simulink model "MicroMouseTemplate"  (R2024a)
settings: Solver=FixedStepAuto  StartTime=0.0  StopTime=10.0  RelTol=1e-3  EnableMultiTasking=on
undefined symbols (not defined in the file or in its folder): samplingTime
settings Model: STM32="{\"DigitalPortWrite\":[{\"ID\":\"MicroMouseTemplate:84:3\"},{\"ID\":\"MicroMouseTemplate:84:4\"},{\"ID\":\"MicroMouseTemplate:84:5\"},{\"ID\":\"MicroMouseTemplate:84:6\"},{\"ID\":\"MicroMouseTemplate:84:7\"},{\"ID\":\"MicroMouseTemplate:84:8\"},{\"ID\":\"MicroMouseTemplate:84:9\"},{\"ID\":\"MicroMouseTemplate:84:10\"},{\"ID\":\"MicroMouseTemplate:160:19\"},{\"ID\":\"MicroMouseTemplate:2479:4\"},{\"ID\":\"MicroMouseTemplate:2479:6\"},{\"ID\":\"MicroMouseTemplate:2479:7\"},{\"ID\":\"MicroMouseTemplate:2479:8\"}],\"PWMOutput\":[{\"ID\":\"MicroMouseTemplate:160:24\"},{\"ID\":\"MicroMouseTemplate:160:25\"}],\"AnalogInput\":{\"ID\":\"MicroMouseTemplate:2357:1\"},\"DigitalPortRead\":[{\"ID\":\"MicroMouseTemplate:2483:3\"},{\"ID\":\"MicroMouseTemplate:2483:4\"}]}"  SimulationMode=external  ExtModeTrigDuration=10  Creator=JesseJabezArendse  LastModifiedBy=Chris Scheepers
settings SolverCC: AllowMultiTaskInputOutput=on  AutoInsertRateTranBlk=on  InsertRTBMode=Never (minimum delay)
settings OptimizationCC: EnhancedBackFolding=on  PassReuseOutputArgsAs=Individual arguments  StateBitsets=on  DataBitsets=on  ZeroExternalMemoryAtStartup=off  ZeroInternalMemoryAtStartup=off  NoFixptDivByZeroProtection=on  MaxStackSize=64  OptimizeBlockOrder=speed  DifferentSizesBufferReuse=on  EfficientTunableParamExpr=on
settings DebuggingCC: MultiTaskCondExecSysMsg=none  ParameterOverflowMsg=none  ParameterPrecisionLossMsg=none  ParameterTunabilityLossMsg=error
settings HardwareCC: ProdBitPerPointer=32  ProdBitPerSizeT=32  ProdBitPerPtrDiffT=32  ProdLargestAtomicInteger=Long  ProdLargestAtomicFloat=Double  ProdWordSize=32  ProdLongLongMode=on  ProdHWDeviceType=ARM Compatible->ARM Cortex  TargetBitPerPointer=64  TargetBitPerSizeT=64  TargetBitPerPtrDiffT=64  TargetLongLongMode=on  TargetIntDivRoundTo=Zero  TargetEndianess=LittleEndian  TargetWordSize=64  TargetHWDeviceType=MATLAB Host
settings ModelReferenceCC: EnableParallelModelReferenceBuilds=on  ParallelModelReferenceMATLABWorkerInit=Copy Base Workspace  SupportModelReferenceSimTargetCustomCode=on
settings SFSimCC: MATLABDynamicMemAlloc=off  SimHardwareAcceleration=native
settings RTWCC: Description=Embedded Coder  SystemTargetFile=ert.tlc  HardwareBoard=STM32L4xx Based  TLCOptions=-p0 -aInlineSetEventsForThisBaseRateFcn=TLC_FALSE -aSuppressMultiTaskScheduler=TLC_FALSE -aRateBasedStepFcn=1  TemplateMakefile=ert_default_tmf  Toolchain=GNU Tools for ARM Embedded Processors  CodeExecutionProfiling=on  CodeProfilingInstrumentation=coarse  GPUComputeCapability=3.5
settings RTWCC: CustomHeaderCode=|
  | #include "MicroMouseProgramming\Core\Inc\IMU.h"
  | #include "MicroMouseProgramming\Core\Inc\CustomWhile.h"
  | #include "MicroMouseProgramming\Core\Inc\Motors.h"
settings RTWCC: CustomInclude=|
  | MicroMouseProgramming\Core\Inc\
  | MicroMouseProgramming\Core\Src\
settings RTWCC: CustomSource=|
  | MicroMouseProgramming\Core\Src\IMU.c
  | MicroMouseProgramming\Core\Src\CustomWhile.c
  | MicroMouseProgramming\Core\Src\Motors.c
settings CodeAppCC: ForceParamTrailComments=on  IgnoreCustomStorageClasses=off  OperatorAnnotations=on  SimulinkDataObjDesc=on  SFDataObjDesc=on  InsertBlockDesc=on
settings ERTTargetCC: CodeReplacementLibrary=ARM Cortex-M  SupportNonFinite=off  SupportComplex=off  SupportContinuousTime=on  ExtModeTransport=3  ExtModeStaticAlloc=on  ExtModeStaticAllocSize=2048  ExtModeMexFile=ext_xcp  ExtModeIntrfLevel=Level2 - Open

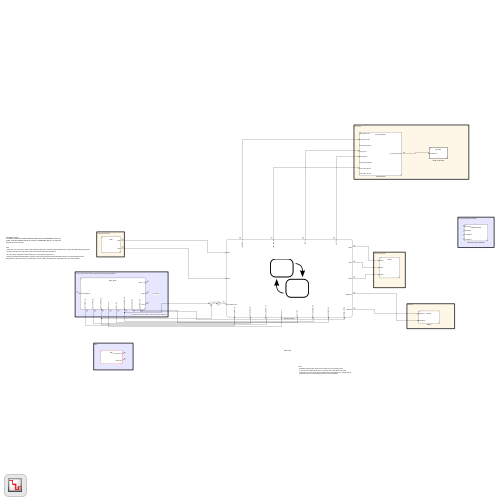
[thumbnail: Simulink's stored preview of the top-level diagram]
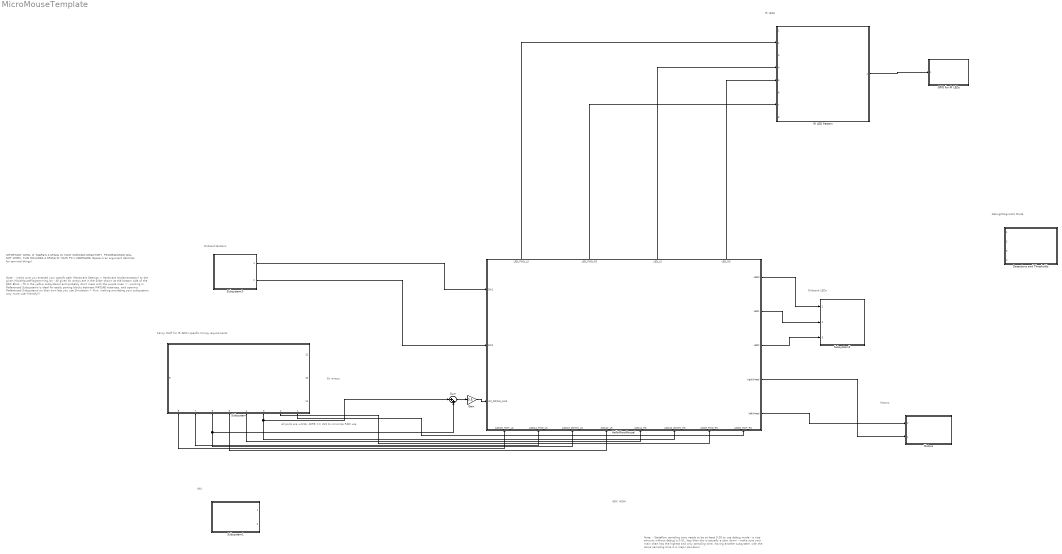
== system MicroMouseTemplate ==
  note: ADC HIGH
  note: IMPORTANT NOTE:
      | IF THERE'S A SPACE IN YOUR WORKING DIRECTORY, PROGRAMMING WILL NOT WORK, THIS INCLUDES A SPACE IN YOUR PC's USERNAME (Space is an argument delimiter for terminal things)
  note: Note:
      | - make sure you entered your specifc path (Hardware Settings > Hardware Implementation) to the given MicroMouseProgramming.ioc
      | - All given 8x arrays are in the order shown at the bottom side of the ADC Block
      |
      | - fill in the yellow subsystems and probably don't mess with the purple ones :)
      | - working in Referenced Subsystems is ideal for easily porting blocks between MATLAB instances, and opening Referenced Subsystems on their own lets you use Simulation > Run, making simulating your subsystems way more user friendly!!!
  note: 8x arrays
  note: all ports are uint16, 4095 == 3V3 to minimize RAM use
  note: IMU
  note: Note:
      | - Stateflow sampling time needs to be at least 0.05 to use debug mode
      | - a nice amount without debug is 0.01, less than this is actually a slow down
      | - make sure your main chart has the highest and only sampling time, having another
      | subsystem with the same sampling time is a major slowdown
  note: Fancy Stuff for IR ADCs specific timing requirements
  note: IR LEDs
  note: Motors
  note: Onboard Buttons
  note: Onboard LEDs
  note: Debug/Diagnostic Mode
  Detections and Thresholds : Subsystem  ReferencedSubsystem=DiagnosticMode
  GPIO for IR LEDs : Subsystem  TreatAsAtomicUnit=on  SystemSampleTime=samplingTime  ReferencedSubsystem=IR_LEDs
  Gain : Gain  Gain=0.5
  HelloMicroMouse! : Stateflow chart  TreatAsAtomicUnit=on  SystemSampleTime=0.05
      settings: PortSchema="{\"entries\":[{\"content\":{\"sides\":[{\"content\":{\"connectorIds\":[\"In11\",\"In10\",\"In3\"]},\"type\":\"ConnectorPlacement.EquallySpacedRectSide\",\"uuid\":\"f52daa4f-6374-42e5-9ef1-0ccc99d09b58\"},{\"content\":{\"connectorIds\":[\"Out5\",\"Out3\",\"Out4\",\"Out2\",\"Out1\"],\"side\":\"RIGHT\"},\"type\":\"ConnectorPlacement.EquallySpacedRectSide\",\"uuid\":\"94b478cc-4dde-45c7-a588-77cf2b43cdb7\"},{\"content\":{\"connectorIds\":[\"Out6\",\"Out7\",\"Out8\",\"Out9\"],\"side\":\"TOP\"},\"type\":\"ConnectorPlacement.EquallySpacedRectSide\",\"uuid\":\"afff2079-ea5c-423e-9722-09c3bbce433b\"},{\"content\":{\"connectorIds\":[\"In1\",\"In2\",\"In4\",\"In5\",\"In6\",\"In7\",\"In8\",\"In9\"],\"side\":\"BOTTOM\"},\"type\":\"ConnectorPlacement.EquallySpacedRectSide\",\"uuid\":\"94e93a1d-795d-41a3-b2d8-d520b2bf47ef\"}]},\"type\":\"ConnectorPlacement.EquallySpacedConnector\",\"uuid\":\"d4d35636-54af-48ac-af70-d56caef5e090\"}],\"packageUris\":[\"http://schema.mathworks.com/mf0/Connector/R2020b\"],\"version\":\"1.0\"}"
  IR LED Pattern : Subsystem  ReferencedSubsystem=IR_LED_Pattern
  Motors : Subsystem  ReferencedSubsystem=Motors
      settings: PortSchema="{\"entries\":[{\"content\":{\"sides\":[{\"content\":{\"connectorIds\":[\"In2\",\"In1\"]},\"type\":\"ConnectorPlacement.EquallySpacedRectSide\",\"uuid\":\"b3741f01-871a-479c-9206-f0581f668097\"},{\"content\":{\"side\":\"RIGHT\"},\"type\":\"ConnectorPlacement.EquallySpacedRectSide\",\"uuid\":\"4e24163a-f10e-40fa-a35f-86add3e4876d\"},{\"content\":{\"side\":\"TOP\"},\"type\":\"ConnectorPlacement.EquallySpacedRectSide\",\"uuid\":\"20b900cb-8f31-42f3-9ac1-0d679ccd8bc0\"}]},\"type\":\"ConnectorPlacement.EquallySpacedConnector\",\"uuid\":\"90358f46-f7a9-48cf-9149-c68081c17f53\"}],\"packageUris\":[\"http://schema.mathworks.com/mf0/Connector/R2020b\"],\"version\":\"1.0\"}"
  Subsystem : Subsystem  ReferencedSubsystem=ADC_Block
      settings: PortSchema="{\"entries\":[{\"content\":{\"sides\":[{\"content\":{},\"type\":\"ConnectorPlacement.EquallySpacedRectSide\",\"uuid\":\"be6b81d5-7a49-4e34-b35f-0c07892094fc\"},{\"content\":{\"connectorIds\":[\"Out1\",\"Out2\",\"Out3\",\"Out4\",\"Out5\",\"Out6\",\"Out7\",\"Out8\"],\"side\":\"RIGHT\"},\"type\":\"ConnectorPlacement.EquallySpacedRectSide\",\"uuid\":\"5e22590a-b7c0-4c63-8de4-8d81fd6c3849\"},{\"content\":{\"connectorIds\":[\"Out12\",\"Out10\",\"Out11\"],\"side\":\"TOP\"},\"type\":\"ConnectorPlacement.EquallySpacedRectSide\",\"uuid\":\"da97636e-cea0-4a10-8fe5-d807f9ee999f\"},{\"content\":{\"connectorIds\":[\"Out9\"],\"side\":\"BOTTOM\"},\"type\":\"ConnectorPlacement.EquallySpacedRectSide\",\"uuid\":\"a593d780-81a8-4730-a8bc-2bbf356cafe4\"}]},\"type\":\"ConnectorPlacement.EquallySpacedConnector\",\"uuid\":\"0bcac921-e51a-4437-9183-315712d0a8c2\"}],\"packageUris\":[\"http://schema.mathworks.com/mf0/Connector/R2020b\"],\"version\":\"1.0\"}"
  Subsystem1 : Subsystem  ReferencedSubsystem=IMU
  Subsystem2 : Subsystem  ReferencedSubsystem=LEDs
  Subsystem3 : Subsystem  ReferencedSubsystem=SWs
  Sum : Sum  Inputs=|++
  wires:
  IR LED Pattern/1 -> GPIO for IR LEDs/1
  Subsystem3/1 -> HelloMicroMouse!/11(SW1)
  HelloMicroMouse!/5(LED0) -> Subsystem2/1
  HelloMicroMouse!/3(LED1) -> Subsystem2/2
  HelloMicroMouse!/4(LED2) -> Subsystem2/3
  Sum/1 -> Gain/1
  Gain/1 -> HelloMicroMouse!/3(init_DOWN_AVG)
  Subsystem3/2 -> HelloMicroMouse!/10(SW2)
  Subsystem/1 -> HelloMicroMouse!/9(ADC8_MOT_RS)
  Subsystem/2 -> HelloMicroMouse!/8(ADC9_FWD_RS)
  Subsystem/3 -> HelloMicroMouse!/7(ADC10_DOWN_RS), Sum/1
  Subsystem/4 -> HelloMicroMouse!/6(ADC11_RS)
  Subsystem/5 -> HelloMicroMouse!/5(ADC12_LS)
  Subsystem/6 -> HelloMicroMouse!/4(ADC13_DOWN_LS), Sum/2
  Subsystem/7 -> HelloMicroMouse!/2(ADC14_FWD_LS)
  Subsystem/8 -> HelloMicroMouse!/1(ADC15_MOT_LS)
  HelloMicroMouse!/2(rightWheel) -> Motors/1
  HelloMicroMouse!/1(leftWheel) -> Motors/2
  HelloMicroMouse!/9(LED_RS) -> IR LED Pattern/5
  HelloMicroMouse!/8(LED_LS) -> IR LED Pattern/4
  HelloMicroMouse!/7(LED_FWD_RS) -> IR LED Pattern/7
  HelloMicroMouse!/6(LED_FWD_LS) -> IR LED Pattern/2

== stateflow chart MicroMouseTemplate/HelloMicroMouse! ==
  state Calibration_Sides [commented out]
    entry:
    counter = 0
    sum_LEFT = 0;
    sum_RIGHT = 0;
    min_LEFT = ADC12_LS;
    min_RIGHT = ADC11_RS;
    during:
    % Collect ADC values for averaging
    if counter < 100
    min_LEFT = min(min_LEFT, ADC12_LS);
    min_RIGHT = min(min_RIGHT, ADC11_RS);
    sum_LEFT = sum_LEFT + min_LEFT;
    sum_RIGHT = sum_RIGHT + min_RIGHT;
    counter = counter + 1;
    else
    % Once 10 samples are collected, calculate the average
    avg_LEFT = (sum_LEFT)/100;
    avg_RIGHT = (sum_RIGHT)/100;
    % Use the averages for calibration or further processing
    init_LEFT = avg_LEFT*0.9;
    init_RIGHT = avg_RIGHT*0.9;
    end
  state CalibrationForward
    entry:
    counter = 0
    sum_FWD_LEFT = 0;
    sum_FWD_RIGHT = 0;
    leftWheel = 75;
    rightWheel = -75;
    LED_FWD_RS = 1;
    LED_FWD_LS = 1;
    during:
    % Collect ADC values for averaging
    leftWheel = leftWheel*(-1);
    rightWheel = rightWheel*(-1);
    if counter < 100
    sum_FWD_LEFT = sum_FWD_LEFT + ADC14_FWD_LS;
    sum_FWD_RIGHT = sum_FWD_RIGHT + ADC9_FWD_RS;
    counter = counter + 1;
    else
    % Once 100 samples are collected, calculate the average
    avg_FWD_LEFT = sum_FWD_LEFT / 100;
    avg_FWD_RIGHT = sum_FWD_RIGHT / 100;
    % Use the averages for calibration or further processing
    init_FWD_LEFT = avg_FWD_LEFT;
    init_FWD_RIGHT = avg_FWD_RIGHT;
    % Optionally: Stop the robot or transition to the next state
    leftWheel = 0;
    rightWheel = 0;
    end
    exit:
    LED_FWD_RS = 0;
    LED_FWD_LS = 0;
  state ButtonPressed3
    entry:
    LED0 = ~LED0;
    LED1 = ~LED1;
    LED2 = ~LED2;
    state Driving
      entry:
      timer = 0;
      during:
      timer = timer +1;
      state Turning_Right_Adjustment
        entry:
        leftWheel = 70;
        rightWheel = 75;
      state Forward
        entry:
        LED0 = false;
        LED1 = false;
        LED2 = false;
        % if abs(ADC13_DOWN_LS - ADC10_DOWN_RS) > down_error
        %    error = true;
        %    check = max(ADC13_DOWN_LS - thresh_down_l, ADC10_DOWN_RS - thresh_down_r)
        %end
        leftWheel = normal_speed_LEFT;
        rightWheel = normal_speed_RIGHT;
        exit:
        % during:
        % curr_d_left = ADC13_DOWN_LS;
        % curr_d_right = ADC10_DOWN_RS;
        % if abs(curr_d_left - curr_d_right) > down_error
        %     error = true;
        %    check = max((curr_d_left - thresh_down_l)*0.8, curr_d_right - thresh_down_r)
        % end
      state Turning_Left_Adjustment
        entry:
        rightWheel = 70;
        leftWheel = 75;
      (default) -> Forward
      Forward -> Turning_Right_Adjustment [order 1] : [ADC13_DOWN_LS > thresh_DOWN_LEFT ]
      Turning_Right_Adjustment -> Forward [order 1] : [ADC10_DOWN_RS<thresh_DOWN_RIGHT && ADC13_DOWN_LS< thresh_DOWN_LEFT]
      Turning_Right_Adjustment -> Turning_Left_Adjustment [order 2] : [ADC10_DOWN_RS > thresh_DOWN_RIGHT]
      Turning_Left_Adjustment -> Turning_Right_Adjustment [order 1] : [ADC13_DOWN_LS > thresh_DOWN_LEFT ]
      Forward -> Turning_Left_Adjustment [order 2] : [ADC10_DOWN_RS > thresh_DOWN_RIGHT]
      Turning_Left_Adjustment -> Forward [order 2] : [ADC10_DOWN_RS<thresh_DOWN_RIGHT && ADC13_DOWN_LS< thresh_DOWN_LEFT]
    state turnLeft
      entry:
      LED0 = true;
      LED1 = false;
      LED2 = false;
      leftWheel = 0;
      rightWheel = 85;
    state CrossDetection
      entry:
      leftWheel = 0;
      rightWheel = 0;
      LED0 = true;
      LED1 = true;
      LED2 = true;
      LEDtimer = 0;
      LEDtimer1 = 0;
      processDone = 0;
      frontClear = false;
      leftClear = false;
      rightClear = false;
      during:
      % Control the LEDs
      LED_LS = 1;
      LED_RS = 1;
      LED_FWD_RS = 0;  % Only turn these on after processing side sensors
      LED_FWD_LS = 0;
      % Update LED timer only once per cycle
      if LEDtimer < 100
      LEDtimer = LEDtimer + 1;
      else
      LEDtimer = 0;
      % Left and right sensor check
      if (ADC12_LS >= thresh_LEFT)
      leftClear = false;
      else
      leftClear = true;
      end
      if (ADC11_RS >= thresh_RIGHT)
      rightClear = false;
      else
      rightClear = true;
      end
      end
      % Now process forward sensors after updating LED states
      LED_LS = 0;
      LED_RS = 0;
      LED_FWD_RS = 1;
      LED_FWD_LS = 1;
      % Check forward sensor readings
      if LEDtimer1 < 100
      LEDtimer1 = LEDtimer1 + 1;
      else
      LEDtimer = 0;
      if ((ADC14_FWD_LS >= thresh_FWD_L) || (ADC9_FWD_RS >= thresh_FWD_R))
      frontClear = false;
      else
      frontClear = true;
      end
      % Crossroad decision
      LED_FWD_RS = 0;
      LED_FWD_LS = 0;
      processDone = 1;
      end
      % Crossroad decision
      if processDone == 1
      if (frontClear && ~rightClear && ~leftClear)
      crossroadCondition = 1;  % Go straight
      elseif (~leftClear && rightClear && ~frontClear)
      crossroadCondition = 2;  % Turn right
      elseif (~rightClear && ~frontClear && leftClear)
      crossroadCondition = 3;  % Turn left
      elseif (~leftClear && ~frontClear && ~rightClear)
      crossroadCondition = 4;  % Turn back
      elseif (rightClear && leftClear && ~frontClear)
      crossroadCondition = 5;  % Turn left
      elseif (leftClear && ~rightClear && frontClear)
      crossroadCondition = 6;  % Turn left
      else
      crossroadCondition = 7;  % Go straight
      end
      else
      end
    state turnRight
      entry:
      LED0 = false;
      LED1 = false;
      LED2 = true;
      leftWheel = 85;
      rightWheel = 0;
    state turnBack
      entry:
      LED0 = false;
      LED1 = true;
      LED2 = false;
      leftWheel =-75;
      rightWheel = 75;
    (default) -> Driving
    turnBack -> Driving : after(2100,msec)
    turnRight -> Driving : after(1300,msec)
    Driving -> CrossDetection : [init_DOWN_AVG<thresh_DOWN_AVG && timer >=25 ]
    CrossDetection -> Driving [order 1] : [crossroadCondition == 7]
    CrossDetection -> Driving [order 2] : [crossroadCondition == 1]
    turnLeft -> Driving : after(1300,msec)
    CrossDetection -> turnLeft [order 3] : [crossroadCondition == 3]
    CrossDetection -> turnLeft [order 5] : [crossroadCondition == 5]
    CrossDetection -> turnLeft [order 7] : [crossroadCondition == 6]
    CrossDetection -> turnRight [order 6] : [crossroadCondition == 2]
    CrossDetection -> turnBack [order 4] : [crossroadCondition == 4]
  state Ready1
    entry:
    % Initial setup
    rightWheel = 0;
    leftWheel = 0;
    LED2 = true;
    LED1 = true;
    LED0 = true;
    LED_FWD_RS = 0;
    LED_FWD_LS = 0;
    LED_LS = 0;
    LED_RS = 0;
    % Calculate thresholds using averaged values
    thresh_DOWN_RIGHT = (init_DOWN_R_LIGHT + init_DOWN_R_DARK)*0.5;
    thresh_DOWN_LEFT = (init_DOWN_L_LIGHT + init_DOWN_L_DARK)*0.5;
    thresh_DOWN_AVG = (init_DOWN_L_DARK+ init_DOWN_R_DARK)*0.5;
    thresh_LEFT = ((init_LEFT_FAR+init_LEFT_CLOSE)*0.5)*0.9;
    thresh_RIGHT =((init_RIGHT_FAR+init_RIGHT_CLOSE)*0.5)*0.9;
    %thresh_FWD_L = ((init_FWD_L_CLOSE+ init_FWD_L_FAR)*0.5)*0.9;
    %thresh_FWD_R =((init_FWD_R_FAR+init_FWD_R_CLOSE)*0.5)*0.9;
    thresh_FWD_L =init_FWD_LEFT;
    thresh_FWD_R = init_FWD_RIGHT;
    thresh_FWD = (thresh_FWD_L + thresh_FWD_R)*0.5;
    % Set normal speeds
    normal_speed_LEFT = 75;
    normal_speed_RIGHT = 75;
  state WaitUntilButtonPressed
    during:
    LED1 = ~LED1;
  state Stop1 [commented out]
    entry:
    LED0 = false;
    LED2 = false;
    leftWheel = 0;
    rightWheel = 0;
    during:
    LED1 = ~LED1;
  state CalibrationDownAndSides
    entry:
    LED1 = true
    LED_LS = 1;
    LED_RS = 1;
    rightWheel = 75;
    leftWheel = -75;
    init_DOWN_R_DARK = ADC10_DOWN_RS;
    init_DOWN_L_DARK = ADC13_DOWN_LS;
    init_DOWN_R_LIGHT = ADC10_DOWN_RS;
    init_DOWN_L_LIGHT = ADC13_DOWN_LS;
    init_LEFT_CLOSE = ADC12_LS;
    init_RIGHT_CLOSE = ADC11_RS;
    init_LEFT_FAR = ADC12_LS;
    init_RIGHT_FAR = ADC11_RS;
    during:
    init_DOWN_R_DARK = min(init_DOWN_R_DARK, ADC10_DOWN_RS);
    init_DOWN_L_DARK = min(init_DOWN_L_DARK, ADC13_DOWN_LS);
    init_DOWN_R_LIGHT = max(init_DOWN_R_LIGHT, ADC10_DOWN_RS);
    init_DOWN_L_LIGHT = max(init_DOWN_L_LIGHT, ADC13_DOWN_LS);
    init_LEFT_CLOSE = max(init_LEFT_CLOSE, ADC12_LS);
    init_RIGHT_CLOSE = max(init_RIGHT_CLOSE, ADC11_RS);
    init_LEFT_FAR = min(init_LEFT_FAR, ADC12_LS);
    init_RIGHT_FAR = min(init_RIGHT_FAR, ADC11_RS);
    exit:
    LED_LS = 0;
    LED_RS = 0;
  (default) -> WaitUntilButtonPressed
  ButtonPressed3 -> Stop1 [commented out] : [ADC14_FWD_LS > init_FWD_LEFT &&  ADC9_FWD_RS > init_FWD_RIGHT]
  Ready1 -> ButtonPressed3 : [SW1]
  WaitUntilButtonPressed -> CalibrationForward : [SW1]
  Stop1 -> ButtonPressed3 [commented out] : [SW2]
  CalibrationForward -> CalibrationDownAndSides : [SW2 && counter==100]
  CalibrationDownAndSides -> Ready1 : after(5,sec)
  data: ADC15_MOT_LS input; ADC14_FWD_LS input; init_DOWN_AVG input; ADC13_DOWN_LS input; ADC12_LS input; ADC11_RS input; ADC10_DOWN_RS input; ADC9_FWD_RS input; ADC8_MOT_RS input; leftWheel output; rightWheel output; LED1 output =false; LED2 output =false; SW2 input; LED0 output =false; SW1 input; init_DOWN_L_LIGHT local; thresh_DOWN_LEFT local; normal_speed_RIGHT local; init_DOWN_R_DARK local; init_DOWN_L_DARK local; thresh_DOWN_RIGHT local; init_DOWN_R_LIGHT local; normal_speed_LEFT local; avg_FWD_LEFT local; counter local; avg_FWD_RIGHT local; sum_FWD_LEFT local uint16; sum_FWD_RIGHT local uint16; avg_LEFT local; avg_RIGHT local; init_LEFT local; init_RIGHT local; sum_LEFT local uint16; sum_RIGHT local uint16; timer local; rightClear local; leftClear local; crossroadCondition local; init_FWD_LEFT local; init_FWD_RIGHT local; thresh_DOWN_AVG local; min_LEFT local; min_RIGHT local; frontClear local boolean; init_FWD_L_LIGHT local; init_FWD_R_DARK local; init_FWD_R_LIGHT local; init_LEFT_DARK local; init_LEFT_LIGHT local; init_RIGHT_DARK local; init_RIGHT_LIGHT local; thresh_FWD_L local; thresh_FWD_R local; thresh_LEFT local; thresh_RIGHT local; init_FWD_L_CLOSE local; init_FWD_L_FAR local; init_FWD_R_CLOSE local; init_FWD_R_FAR local; init_LEFT_CLOSE local; init_LEFT_FAR local; init_RIGHT_CLOSE local; init_RIGHT_FAR local; thresh_FWD local; leftWallDetectCounter local; consecutiveThreshold local; rightWallDetectCounter local; frontWallDetectCounter local; waitTime local; LED_FWD_LS output; LED_FWD_RS output; LED_LS output; LED_RS output; LEDtimer local; processDone local; LEDtimer1 local
